simulink model "problem_1"  (R2020b)
settings: Solver=VariableStepAuto  StartTime=0.0  StopTime=10.0  RelTol=1e-3
settings Model: Creator=hp  LastModifiedBy=hp

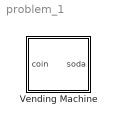
== system problem_1 ==
  Vending Machine : Stateflow chart  TreatAsAtomicUnit=on

== stateflow chart problem_1/Vending Machine ==
  state recived_0
  state recived_1
  (default) -> recived_0
  recived_0 -> recived_1 : [coin==1]{soda=0}
  recived_1 -> recived_0
  data: coin input; soda output
